simulink model "Beamform_Array"  (R2019b)
settings: Solver=VariableStepAuto  StartTime=0.0  StopTime=10.0  RelTol=1e-3
settings Model: Creator=toons  LastModifiedBy=toons
settings DataIOCC: ReturnWorkspaceOutputs=off
settings DebuggingCC: ArithmeticOperatorsInVariantConditions=warning
settings SFSimCC: CustomCodeUndefinedFunction=UseInterfaceOnly

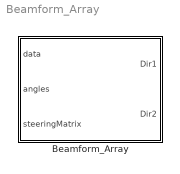
== system Beamform_Array ==
  Beamform_Array : Subsystem

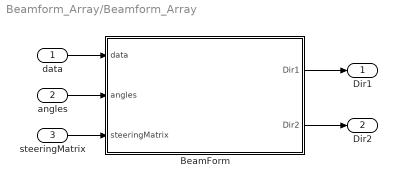
== system Beamform_Array/Beamform_Array ==
  data : Inport
  angles : Inport  Port=2
  steeringMatrix : Inport  Port=3
  BeamForm : MATLAB Function  TreatAsAtomicUnit=on
  Dir1 : Outport
  Dir2 : Outport  Port=2
  wires:
  data/1 -> BeamForm/1(data)
  BeamForm/1(Dir1) -> Dir1/1
  angles/1 -> BeamForm/2(angles)
  BeamForm/2(Dir2) -> Dir2/1
  steeringMatrix/1 -> BeamForm/3(steeringMatrix)

== matlab function Beamform_Array/BeamForm ==
  data: data input; Dir1 output; angles input; steeringMatrix input; Dir2 output
function [Dir1, Dir2] = BeamForm(data, angles, steeringMatrix)
%BeamForm Beamform execution block
   powerAngles = appBeamformer('Frequency domain', 'Wide', data, ...
       steeringMatrix, angles, 'Delay and Sum', 'Dense Array', 1);
   [~, index] = max(powerAngles);
   Dir1 = angles(1,index);
   Dir2 = angles(2,index);
end
